simulink model "airbag_statflow"  (R2015b)
settings: Solver=FixedStepAuto  StartTime=0.0  StopTime=inf  FixedStep=0.1  RelTol=1e-3
settings Model: Creator=scco1019  LastModifiedBy=scco1019

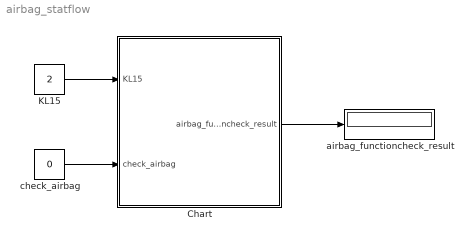
== system airbag_statflow ==
  Chart : Stateflow chart  TreatAsAtomicUnit=on
  KL15 : Constant  Value=2
  airbag_functioncheck_result : Display
  check_airbag : Constant  Value=0
  wires:
  KL15/1 -> Chart/1(KL15)
  check_airbag/1 -> Chart/2(check_airbag)
  Chart/1(airbag_functioncheck_result) -> airbag_functioncheck_result/1

== stateflow chart airbag_statflow/Chart ==
  (default) -> (junction 5)
  (junction 5) -> (junction 9) [order 2] : {airbag_functioncheck_result=1}
  (junction 5) -> (junction 7) [order 1] : [((KL15>1&&KL15<5))&&(check_airbag==0)]
  (junction 7) -> (junction 11) : {airbag_functioncheck_result=0}
  data: KL15 input; airbag_functioncheck_result output; check_airbag input
